simulink model "Trans"  (R2017a)
settings: Solver=ode15s  StartTime=0.0  StopTime=10  MaxStep=1e-3  RelTol=1e-8  AbsTol=1e-6
values from neighbouring files (symbols this model uses):
  r1 = 0.25    [parameters.m]
  rp2 = 0.134    [parameters.m]
  wb = 2*pi*f    (= 376.991118431)    [parameters.m]
  xl1 = 0.056    [parameters.m]
  xml = 708.8    [parameters.m]
  xpl2 = 0.056    [parameters.m]
settings Model: Creator=Omid  LastModifiedBy=Omid
settings DataIOCC: SaveFormat=Array  SignalLoggingSaveFormat=ModelDataLogs  SaveOutput=off  SaveTime=off
settings OptimizationCC: BlockReduction=off  BooleanDataType=off
settings DebuggingCC: SaveWithParameterizedLinksMsg=none  UnderspecifiedInitializationDetection=Classic  MergeDetectMultiDrivingBlocksExec=none  SignalResolutionControl=TryResolveAllWithWarning  MultiTaskDSMMsg=warning  MultiTaskCondExecSysMsg=none
settings HardwareCC: TargetUnknown=on
settings ModelReferenceCC: PropagateSignalLabelsOutOfModel=off
settings SFSimCC: SimUseLocalCustomCode=on
settings RTWCC: RTWUseLocalCustomCode=on

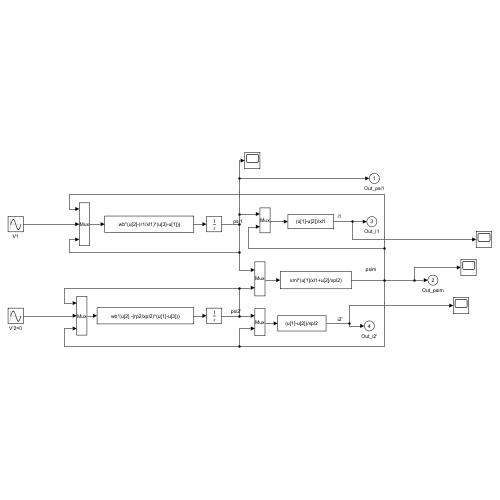
[thumbnail: Simulink's stored preview of the top-level diagram]
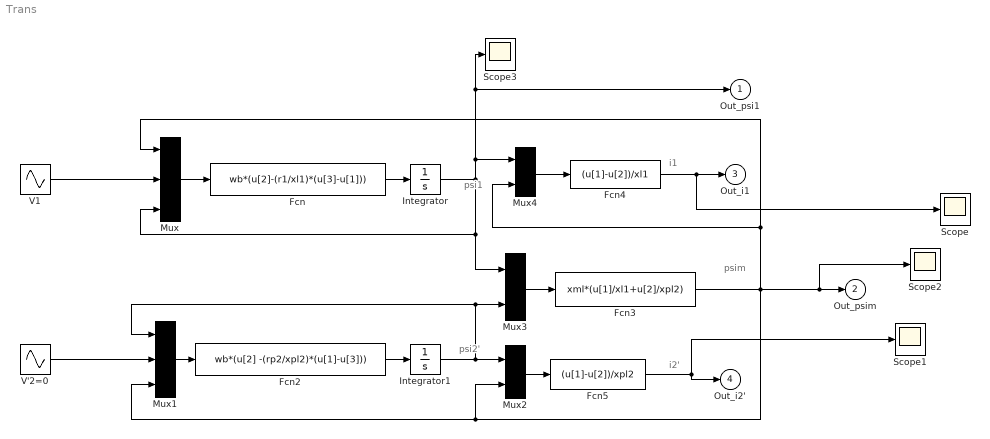
== system Trans ==
  note: i2'
  note: psi1
  note: psi2'
  note: i1
  note: psim
  Fcn : Fcn  Expr=wb*(u[2]-(r1/xl1)*(u[3]-u[1]))
  Fcn2 : Fcn  Expr=wb*(u[2] -(rp2/xpl2)*(u[1]-u[3]))
  Fcn3 : Fcn  Expr=xml*(u[1]/xl1+u[2]/xpl2)
  Fcn4 : Fcn  Expr=(u[1]-u[2])/xl1
  Fcn5 : Fcn  Expr=(u[1]-u[2])/xpl2
  Integrator : Integrator
  Integrator1 : Integrator
  Mux : Mux  Inputs=3
  Mux1 : Mux  Inputs=3
  Mux2 : Mux  Inputs=2
  Mux3 : Mux  Inputs=2
  Mux4 : Mux  Inputs=2
  Scope{,1..3} (4 alike) : Scope
  V'2=0 : Sin  Amplitude=0  SampleTime=0
  V1 : Sin  Amplitude=120  Frequency=120*pi  Samples=60  SampleTime=0
  Out_psi1 : Outport  InitialOutput=0
  Out_psim : Outport  Port=2  InitialOutput=0
  Out_i1 : Outport  Port=3  InitialOutput=0
  Out_i2' : Outport  Port=4  InitialOutput=0
  wires:
  V1/1 -> Mux/2
  Mux/1 -> Fcn/1
  Fcn/1 -> Integrator/1
  Fcn2/1 -> Integrator1/1
  Integrator/1 -> Mux3/1, Mux/3, Scope3/1, Out_psi1/1, Mux4/1
  Fcn3/1 -> Mux/1, Mux4/2, Scope2/1, Out_psim/1, Mux1/3, Mux2/2
  Mux1/1 -> Fcn2/1
  V'2=0/1 -> Mux1/2
  Integrator1/1 -> Mux3/2, Mux1/1, Mux2/1
  Mux2/1 -> Fcn5/1
  Fcn5/1 -> Scope1/1, Out_i2'/1
  Mux3/1 -> Fcn3/1
  Mux4/1 -> Fcn4/1
  Fcn4/1 -> Scope/1, Out_i1/1
